simulink library "rev1CyclopsLib"  (R2021a)
settings: Solver=VariableStepAuto  StartTime=0.0  StopTime=10.0  RelTol=1e-3
values from neighbouring files (symbols this model uses):
  D_32 = [ 1,  4,  8,  2, 16]    [rev1BB_setup.m]
  trFarrowTaps = 4    [rev1BB_setup.m]
  trTappedDelayLen = trTappedDelayBase+trFarrowTaps    (= 44)    [rev1BB_setup.m]
  W_32 = [-1,  1, -1,  1, -1]    [rev1BB_setup.m]
libraries: $bdroot x8, simulink x1
settings Model: Creator=cyarp  LastModifiedBy=cyarp
settings SolverCC: AlgebraicLoopSolver=TrustRegion
settings DebuggingCC: SFMachineParentedDataDiag=warning

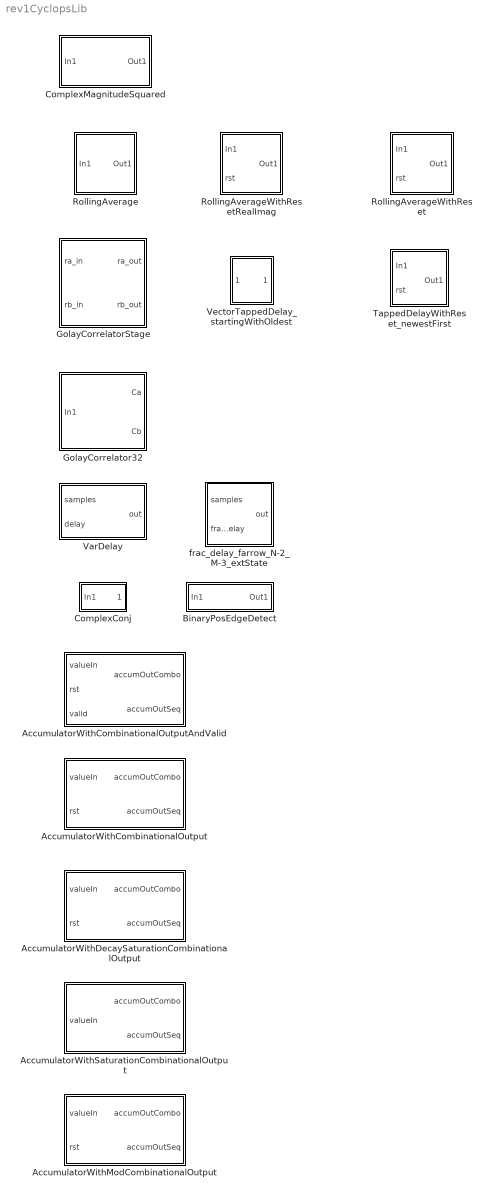
== system rev1CyclopsLib ==
  AccumulatorWithCombinationalOutput : Subsystem  mask(Accumulator with Combinational Output){ResetVal=0}
      mask prompts: ResetVal "Reset Value"
  AccumulatorWithCombinationalOutputAndValid : Subsystem  mask(Accumulator with Combinational Output){ResetVal=0}
      mask prompts: ResetVal "Reset Value"
  AccumulatorWithDecaySaturationCombinationalOutput : Subsystem  mask(Accumulator with Combinational Output){ResetVal=0, Decay=.99, SatUp=10, SatDown=-10}
      mask prompts: ResetVal "Reset Value"; Decay "Decay Multiplier"; SatUp "Saturate Upper Bound"; SatDown "Saturate Lower Bound"
  AccumulatorWithModCombinationalOutput : Subsystem  mask(Accumulator with Combinational Output){ResetVal=0, ModBy=2*pi}
      mask prompts: ResetVal "Reset Value"; ModBy "Mod By"
  AccumulatorWithSaturationCombinationalOutput : Subsystem  mask(Accumulator with Combinational Output){SatUp=10, SatDown=-10}
      mask prompts: SatUp "Saturate Upper Bound"; SatDown "Saturate Lower Bound"
  BinaryPosEdgeDetect : Subsystem
  ComplexConj : Subsystem
  ComplexMagnitudeSquared : Subsystem
  GolayCorrelator32 : Subsystem  mask{sampPerSym=1}
      mask prompts: sampPerSym "Samples Per Symbol"
      mask DialogControl Control2 Prompt: If running in symbol domain, set Samples Per Symbol to 1
  GolayCorrelatorStage : Subsystem  mask{dSub=0, wSub=0}
      mask prompts: dSub "D Paramerer"; wSub "W Parameter"
  RollingAverage : Subsystem  mask{averagingSamples=16}
      mask prompts: averagingSamples "Samples to Average Over"
  RollingAverageWithReset : Subsystem  mask{averagingSamples=16}
      mask prompts: averagingSamples "Samples to Average Over"
  RollingAverageWithResetRealImag : Subsystem  mask{averagingSamples=16}
      mask prompts: averagingSamples "Samples to Average Over"
  TappedDelayWithReset_newestFirst : Subsystem  mask{Depth=2, RstVal=0}
      mask prompts: RstVal "Reset Value"
  VarDelay : Subsystem
  VectorTappedDelay_startingWithOldest : Subsystem  mask{VecLen=2, Depth=3, InitCond=0}
      mask prompts: VecLen "Vector Length"; InitCond "Initial Conditions"
  frac_delay_farrow_N-2_M-3_extState : Subsystem

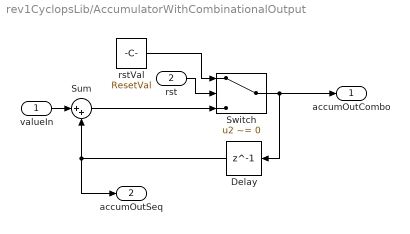
== system rev1CyclopsLib/AccumulatorWithCombinationalOutput ==
  valueIn : Inport
  rst : Inport  Port=2
  Delay : Delay  DelayLength=1  InitialCondition=ResetVal
  Sum : Sum  Inputs=|++  OutDataTypeStr=Inherit: Same as first input
  Switch : Switch  Criteria=u2 ~= 0
  rstVal : Constant  Value=ResetVal  OutDataTypeStr=Inherit: Inherit via back propagation
  accumOutCombo : Outport
  accumOutSeq : Outport  Port=2
  wires:
  rstVal/1 -> Switch/1
  rst/1 -> Switch/2
  Switch/1 -> Delay/1, accumOutCombo/1
  valueIn/1 -> Sum/1
  Delay/1 -> accumOutSeq/1, Sum/2
  Sum/1 -> Switch/3

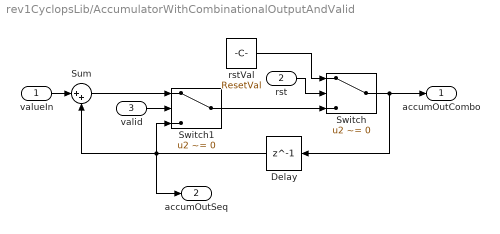
== system rev1CyclopsLib/AccumulatorWithCombinationalOutputAndValid ==
  valueIn : Inport
  rst : Inport  Port=2
  valid : Inport  Port=3  OutDataTypeStr=boolean
  Delay : Delay  DelayLength=1  InitialCondition=ResetVal
  Sum : Sum  Inputs=|++  OutDataTypeStr=Inherit: Same as first input
  Switch : Switch  Criteria=u2 ~= 0
  Switch1 : Switch  Criteria=u2 ~= 0
  rstVal : Constant  Value=ResetVal  OutDataTypeStr=Inherit: Inherit via back propagation
  accumOutCombo : Outport
  accumOutSeq : Outport  Port=2
  wires:
  Sum/1 -> Switch1/1
  rstVal/1 -> Switch/1
  rst/1 -> Switch/2
  Switch1/1 -> Switch/3
  valid/1 -> Switch1/2
  Switch/1 -> Delay/1, accumOutCombo/1
  valueIn/1 -> Sum/1
  Delay/1 -> accumOutSeq/1, Switch1/3, Sum/2

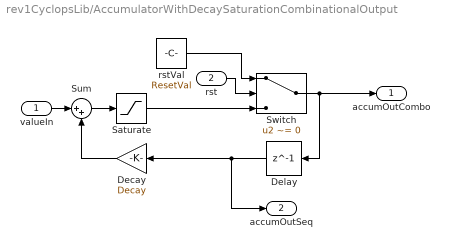
== system rev1CyclopsLib/AccumulatorWithDecaySaturationCombinationalOutput ==
  valueIn : Inport
  rst : Inport  Port=2
  Decay : Gain  Gain=Decay
  Delay : Delay  DelayLength=1  InitialCondition=ResetVal
  Saturate : Saturate  UpperLimit=SatUp  LowerLimit=SatDown
  Sum : Sum  Inputs=|++  OutDataTypeStr=Inherit: Same as first input
  Switch : Switch  Criteria=u2 ~= 0
  rstVal : Constant  Value=ResetVal  OutDataTypeStr=Inherit: Inherit via back propagation
  accumOutCombo : Outport
  accumOutSeq : Outport  Port=2
  wires:
  rstVal/1 -> Switch/1
  rst/1 -> Switch/2
  Switch/1 -> Delay/1, accumOutCombo/1
  valueIn/1 -> Sum/1
  Delay/1 -> accumOutSeq/1, Decay/1
  Sum/1 -> Saturate/1
  Decay/1 -> Sum/2
  Saturate/1 -> Switch/3

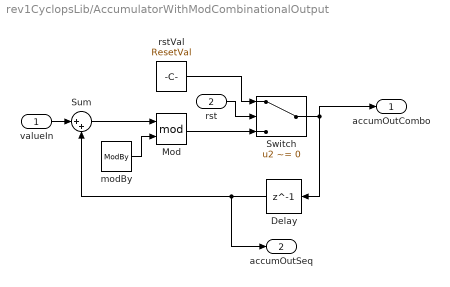
== system rev1CyclopsLib/AccumulatorWithModCombinationalOutput ==
  valueIn : Inport
  rst : Inport  Port=2
  Delay : Delay  DelayLength=1  InitialCondition=ResetVal
  Mod : Math  Operator=mod  SaturateOnIntegerOverflow=on
  Sum : Sum  Inputs=|++  OutDataTypeStr=Inherit: Same as first input
  Switch : Switch  Criteria=u2 ~= 0
  modBy : Constant  Value=ModBy  OutDataTypeStr=Inherit: Inherit via back propagation
  rstVal : Constant  Value=ResetVal  OutDataTypeStr=Inherit: Inherit via back propagation
  accumOutCombo : Outport
  accumOutSeq : Outport  Port=2
  wires:
  rstVal/1 -> Switch/1
  rst/1 -> Switch/2
  Switch/1 -> accumOutCombo/1, Delay/1
  valueIn/1 -> Sum/1
  Sum/1 -> Mod/1
  Delay/1 -> Sum/2, accumOutSeq/1
  Mod/1 -> Switch/3
  modBy/1 -> Mod/2

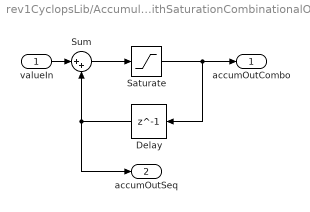
== system rev1CyclopsLib/AccumulatorWithSaturationCombinationalOutput ==
  valueIn : Inport
  Delay : Delay  DelayLength=1
  Saturate : Saturate  UpperLimit=SatUp  LowerLimit=SatDown
  Sum : Sum  Inputs=|++  OutDataTypeStr=Inherit: Same as first input
  accumOutCombo : Outport
  accumOutSeq : Outport  Port=2
  wires:
  Saturate/1 -> accumOutCombo/1, Delay/1
  valueIn/1 -> Sum/1
  Sum/1 -> Saturate/1
  Delay/1 -> Sum/2, accumOutSeq/1

== system rev1CyclopsLib/BinaryPosEdgeDetect ==
  In1 : Inport
  AND : Logic  IconShape=distinctive  AllPortsSameDT=off  OutDataTypeStr=boolean
  Delay : Delay  DelayLength=1
  NOT : Logic  Operator=NOT  IconShape=distinctive  AllPortsSameDT=off  OutDataTypeStr=boolean
  Out1 : Outport
  wires:
  NOT/1 -> AND/2
  AND/1 -> Out1/1
  Delay/1 -> NOT/1
  In1/1 -> AND/1, Delay/1

== system rev1CyclopsLib/ComplexConj ==
  In1 : Inport
  Complex to Real-Imag : ComplexToRealImag
  Gain : Gain  Gain=-1
  Real-Imag to Complex : RealImagToComplex
  Out1 : Outport
  wires:
  Gain/1 -> Real-Imag to Complex/2
  Complex to Real-Imag/2 -> Gain/1
  Complex to Real-Imag/1 -> Real-Imag to Complex/1
  Real-Imag to Complex/1 -> Out1/1
  In1/1 -> Complex to Real-Imag/1

== system rev1CyclopsLib/ComplexMagnitudeSquared ==
  In1 : Inport
  Complex to Real-Imag : ComplexToRealImag
  Product : Product  OutDataTypeStr=Inherit: Same as first input
  Product1 : Product  OutDataTypeStr=Inherit: Same as first input
  Sum : Sum  Inputs=+|+  OutDataTypeStr=Inherit: Same as first input
  Out1 : Outport
  wires:
  In1/1 -> Complex to Real-Imag/1
  Sum/1 -> Out1/1
  Product1/1 -> Sum/2
  Product/1 -> Sum/1
  Complex to Real-Imag/2 -> Product1/1, Product1/2
  Complex to Real-Imag/1 -> Product/1, Product/2

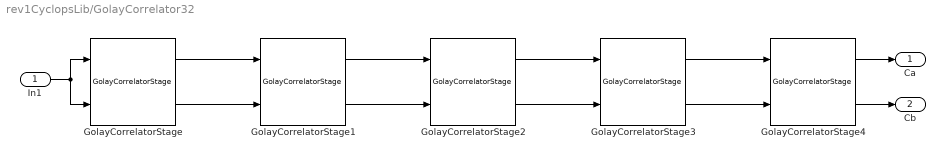
== system rev1CyclopsLib/GolayCorrelator32 ==
  In1 : Inport
  GolayCorrelatorStage : $bdroot/GolayCorrelatorStage  dSub=D_32(1)*sampPerSym  wSub=W_32(1)
  GolayCorrelatorStage1 : $bdroot/GolayCorrelatorStage  dSub=D_32(2)*sampPerSym  wSub=W_32(2)
  GolayCorrelatorStage2 : $bdroot/GolayCorrelatorStage  dSub=D_32(3)*sampPerSym  wSub=W_32(3)
  GolayCorrelatorStage3 : $bdroot/GolayCorrelatorStage  dSub=D_32(4)*sampPerSym  wSub=W_32(4)
  GolayCorrelatorStage4 : $bdroot/GolayCorrelatorStage  dSub=D_32(5)*sampPerSym  wSub=W_32(5)
  Ca : Outport
  Cb : Outport  Port=2
  wires:
  GolayCorrelatorStage3/1 -> GolayCorrelatorStage4/1
  GolayCorrelatorStage3/2 -> GolayCorrelatorStage4/2
  GolayCorrelatorStage2/2 -> GolayCorrelatorStage3/2
  GolayCorrelatorStage2/1 -> GolayCorrelatorStage3/1
  GolayCorrelatorStage1/2 -> GolayCorrelatorStage2/2
  GolayCorrelatorStage1/1 -> GolayCorrelatorStage2/1
  In1/1 -> GolayCorrelatorStage/1, GolayCorrelatorStage/2
  GolayCorrelatorStage4/2 -> Cb/1
  GolayCorrelatorStage4/1 -> Ca/1
  GolayCorrelatorStage/2 -> GolayCorrelatorStage1/2
  GolayCorrelatorStage/1 -> GolayCorrelatorStage1/1

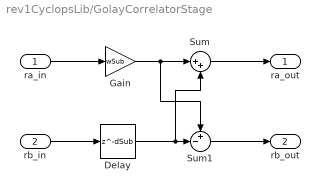
== system rev1CyclopsLib/GolayCorrelatorStage ==
  ra_in : Inport
  rb_in : Inport  Port=2
  Delay : Delay  DelayLength=dSub
  Gain : Gain  Gain=wSub  OutDataTypeStr=Inherit: Same as input
  Sum : Sum  Inputs=|++  OutDataTypeStr=Inherit: Same as first input
  Sum1 : Sum  Inputs=+-|  OutDataTypeStr=Inherit: Same as first input
  ra_out : Outport
  rb_out : Outport  Port=2
  wires:
  rb_in/1 -> Delay/1
  Sum1/1 -> rb_out/1
  Sum/1 -> ra_out/1
  Delay/1 -> Sum1/2, Sum/2
  Gain/1 -> Sum/1, Sum1/1
  ra_in/1 -> Gain/1

== system rev1CyclopsLib/RollingAverage ==
  In1 : Inport
  Averaging Filter FIR : DiscreteFir  Coefficients=ones(1, averagingSamples)./averagingSamples
  Out1 : Outport
  wires:
  Averaging Filter FIR/1 -> Out1/1
  In1/1 -> Averaging Filter FIR/1

== system rev1CyclopsLib/RollingAverageWithReset ==
  In1 : Inport
  rst : Inport  Port=2
  Coefs : Constant  Value=ones(1, averagingSamples)./averagingSamples  OutDataTypeStr=Inherit: Inherit via back propagation
  Dot Product : DotProduct  InputSameDT=on  OutDataTypeStr=Inherit: Inherit via internal rule
  TappedDelayWithReset_newestFirst : $bdroot/TappedDelayWithReset_newestFirst  Depth=averagingSamples  RstVal=0
  Out1 : Outport
  wires:
  Coefs/1 -> Dot Product/2
  Dot Product/1 -> Out1/1
  TappedDelayWithReset_newestFirst/1 -> Dot Product/1
  rst/1 -> TappedDelayWithReset_newestFirst/2
  In1/1 -> TappedDelayWithReset_newestFirst/1

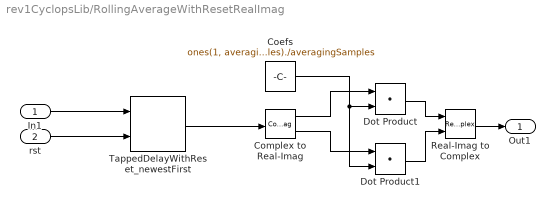
== system rev1CyclopsLib/RollingAverageWithResetRealImag ==
  In1 : Inport
  rst : Inport  Port=2
  Coefs : Constant  Value=ones(1, averagingSamples)./averagingSamples  OutDataTypeStr=Inherit: Inherit via back propagation
  Complex to Real-Imag : ComplexToRealImag
  Dot Product : DotProduct  InputSameDT=on  OutDataTypeStr=Inherit: Inherit via internal rule
  Dot Product1 : DotProduct  InputSameDT=on  OutDataTypeStr=Inherit: Inherit via internal rule
  Real-Imag to Complex : RealImagToComplex
  TappedDelayWithReset_newestFirst : $bdroot/TappedDelayWithReset_newestFirst  Depth=averagingSamples  RstVal=0
  Out1 : Outport
  wires:
  Complex to Real-Imag/1 -> Dot Product/1
  Complex to Real-Imag/2 -> Dot Product1/1
  Coefs/1 -> Dot Product1/2, Dot Product/2
  Dot Product/1 -> Real-Imag to Complex/1
  Dot Product1/1 -> Real-Imag to Complex/2
  Real-Imag to Complex/1 -> Out1/1
  TappedDelayWithReset_newestFirst/1 -> Complex to Real-Imag/1
  In1/1 -> TappedDelayWithReset_newestFirst/1
  rst/1 -> TappedDelayWithReset_newestFirst/2

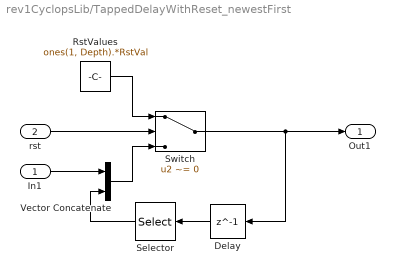
== system rev1CyclopsLib/TappedDelayWithReset_newestFirst ==
  In1 : Inport  PortDimensions=1
  rst : Inport  Port=2
  Delay : Delay  DelayLength=1
  RstValues : Constant  Value=ones(1, Depth).*RstVal  OutDataTypeStr=Inherit: Inherit via back propagation
  Selector : Selector  IndexMode=Zero-based  InputPortWidth=Depth  IndexOptions=Starting index (dialog)  Indices=0  OutputSizes=Depth-1
  Switch : Switch  Criteria=u2 ~= 0
  Vector Concatenate : Concatenate
  Out1 : Outport  PortDimensions=[Depth]
  wires:
  rst/1 -> Switch/2
  RstValues/1 -> Switch/1
  Vector Concatenate/1 -> Switch/3
  Delay/1 -> Selector/1
  In1/1 -> Vector Concatenate/1
  Switch/1 -> Delay/1, Out1/1
  Selector/1 -> Vector Concatenate/2

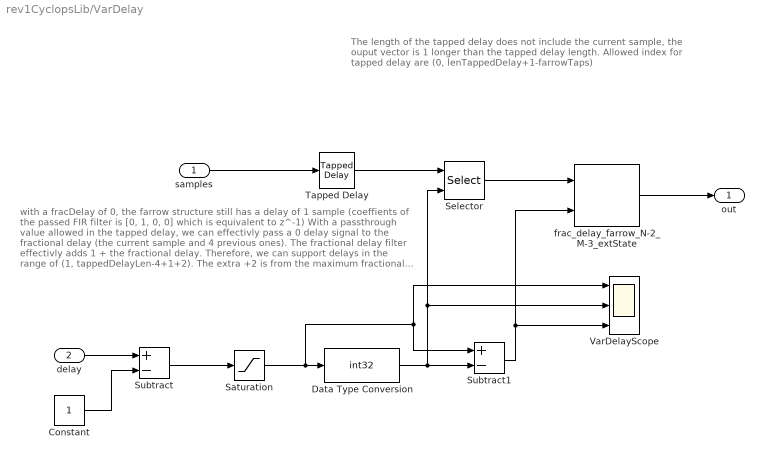
== system rev1CyclopsLib/VarDelay ==
  note: The length of the tapped delay does not include the current sample,
      | the ouput vector is 1 longer than the tapped delay length.
      |
      | Allowed index for tapped delay are (0, lenTappedDelay+1-farrowTaps)
  note: with a fracDelay of 0, the farrow structure still has a delay of 1 sample
      | (coeffients of the passed FIR filter is [0, 1, 0, 0] which is equivalent to z^-1)
      | With a passthrough value allowed in the tapped delay, we can effectivly
      | pass a 0 delay signal to the fractional delay (the current sample and 4 previous
      | ones).  The fractional delay filter effectivly adds 1 + the fractional delay.
      | Therefore, we can support delays in the range of (1, tappedDelayLen-4+1+2).
      | The extra +2 is from the maximum fractional delay
  samples : Inport
  delay : Inport  Port=2  OutDataTypeStr=single
  Constant : Constant  OutDataTypeStr=Inherit: Inherit via back propagation
  Data Type Conversion : DataTypeConversion  OutDataTypeStr=int32
  Saturation : Saturate  UpperLimit=trTappedDelayLen+1-trFarrowTaps  LowerLimit=0  LinearizeAsGain=off
  Selector : Selector  IndexMode=Zero-based  InputPortWidth=trTappedDelayLen+1  IndexOptions=Starting index (port)  Indices=[1 3]  OutputSizes=trFarrowTaps
  Subtract : Sum  Inputs=+-  OutDataTypeStr=Inherit: Same as first input
  Subtract1 : Sum  Inputs=+-  OutDataTypeStr=Inherit: Same as first input
  Tapped Delay : simulink/Discrete/Tapped Delay  vinit=0.0  samptime=-1  NumDelays=trTappedDelayLen  DelayOrder=Newest  includeCurrent=on
  VarDelayScope : Scope  NumInputPorts=3
  frac_delay_farrow_N-2_M-3_extState : $bdroot/frac_delay_farrow_N-2_M-3_extState  SystemSampleTime=-1  Latency=0  AutoFrameSizeCalculation=off
  out : Outport  VectorParamsAs1DForOutWhenUnconnected=off
  wires:
  frac_delay_farrow_N-2_M-3_extState/1 -> out/1
  samples/1 -> Tapped Delay/1
  Tapped Delay/1 -> Selector/1
  Selector/1 -> frac_delay_farrow_N-2_M-3_extState/1
  delay/1 -> Subtract/1
  Subtract/1 -> Saturation/1
  Saturation/1 -> VarDelayScope/1, Subtract1/1, Data Type Conversion/1
  Constant/1 -> Subtract/2
  Subtract1/1 -> frac_delay_farrow_N-2_M-3_extState/2, VarDelayScope/3
  Data Type Conversion/1 -> Subtract1/2, Selector/2, VarDelayScope/2

== system rev1CyclopsLib/VectorTappedDelay_startingWithOldest ==
  In1 : Inport  PortDimensions=[VecLen]
  Delay6 : Delay  DelayLength=1  InitialCondition=InitCond
  Matrix Concatenate : Concatenate  Mode=Multidimensional array  ConcatenateDimension=2
  Selector : Selector  NumberOfDimensions=2  InputPortWidth=3  IndexOptions=Starting index (dialog),Starting index (dialog)  Indices=1,2  OutputSizes=VecLen,Depth-1
  Out1 : Outport  PortDimensions=[VecLen, Depth]
  wires:
  Selector/1 -> Matrix Concatenate/1
  Matrix Concatenate/1 -> Delay6/1, Out1/1
  Delay6/1 -> Selector/1
  In1/1 -> Matrix Concatenate/2

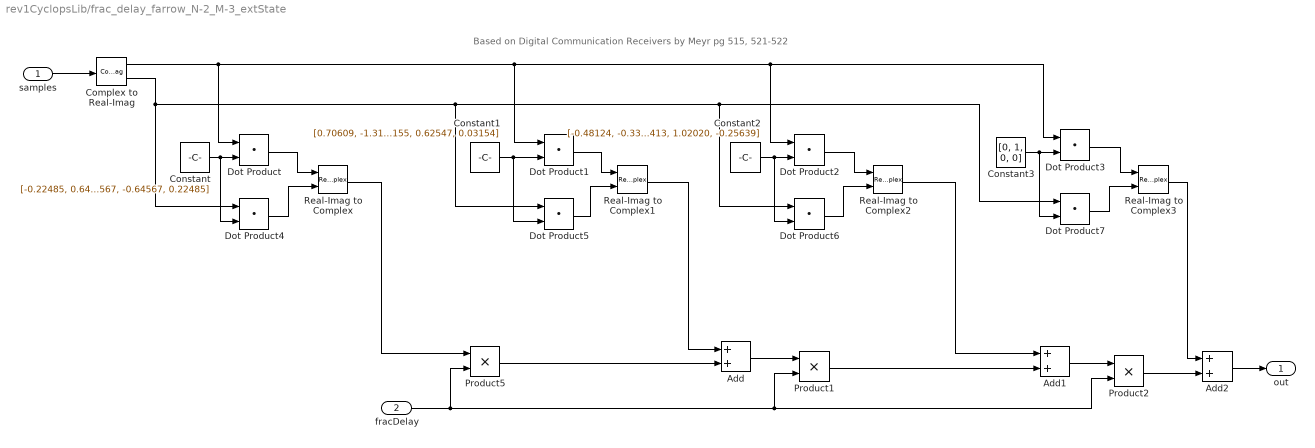
== system rev1CyclopsLib/frac_delay_farrow_N-2_M-3_extState ==
  note: Based on Digital Communication Receivers by Meyr pg 515, 521-522
  samples : Inport  PortDimensions=4
  fracDelay : Inport  Port=2
  Add : Sum
  Add1 : Sum
  Add2 : Sum
  Complex to Real-Imag : ComplexToRealImag
  Constant : Constant  Value=[-0.22485, 0.64567, -0.64567, 0.22485]  OutDataTypeStr=Inherit: Inherit via back propagation
  Constant1 : Constant  Value=[0.70609, -1.31155, 0.62547, 0.03154]  OutDataTypeStr=Inherit: Inherit via back propagation
  Constant2 : Constant  Value=[-0.48124, -0.33413, 1.02020, -0.25639]  OutDataTypeStr=Inherit: Inherit via back propagation
  Constant3 : Constant  Value=[0, 1, 0, 0]  OutDataTypeStr=Inherit: Inherit via back propagation
  Dot Product{,1..7} (8 alike) : DotProduct  InputSameDT=on  OutDataTypeStr=Inherit: Inherit via internal rule
  Product1 : Product  OutDataTypeStr=Inherit: Same as first input
  Product2 : Product  OutDataTypeStr=Inherit: Same as first input
  Product5 : Product  OutDataTypeStr=Inherit: Same as first input
  Real-Imag to Complex{,1..3} (4 alike) : RealImagToComplex
  out : Outport  VectorParamsAs1DForOutWhenUnconnected=off
  wires:
  Dot Product7/1 -> Real-Imag to Complex3/2
  Dot Product3/1 -> Real-Imag to Complex3/1
  Real-Imag to Complex2/1 -> Add1/1
  Dot Product6/1 -> Real-Imag to Complex2/2
  Dot Product2/1 -> Real-Imag to Complex2/1
  Real-Imag to Complex1/1 -> Add/1
  Dot Product5/1 -> Real-Imag to Complex1/2
  Dot Product1/1 -> Real-Imag to Complex1/1
  Dot Product4/1 -> Real-Imag to Complex/2
  Dot Product/1 -> Real-Imag to Complex/1
  Constant3/1 -> Dot Product3/2, Dot Product7/2
  Complex to Real-Imag/2 -> Dot Product5/1, Dot Product7/1, Dot Product6/1, Dot Product4/1
  samples/1 -> Complex to Real-Imag/1
  Constant2/1 -> Dot Product2/2, Dot Product6/2
  Constant1/1 -> Dot Product5/2, Dot Product1/2
  Constant/1 -> Dot Product/2, Dot Product4/2
  fracDelay/1 -> Product2/2, Product1/2, Product5/2
  Product1/1 -> Add1/2
  Product2/1 -> Add2/2
  Add/1 -> Product1/1
  Real-Imag to Complex/1 -> Product5/1
  Add2/1 -> out/1
  Add1/1 -> Product2/1
  Complex to Real-Imag/1 -> Dot Product3/1, Dot Product2/1, Dot Product1/1, Dot Product/1
  Real-Imag to Complex3/1 -> Add2/1
  Product5/1 -> Add/2
